simulink model "Simulation_3DOF01"  (R2024a)
settings: Solver=ode4  StartTime=initial_time  StopTime=final_time  FixedStep=timestep  RelTol=1e-3
values from neighbouring files (symbols this model uses):
  flight_path_angle_0 = flight_path_angle_0 * (pi / 180)    (= 0.0523598775598)    [Constants_3DOF.m]
  heading_angle_0 = heading_angle_0 * (pi/180)    (= 0.349065850399)    [Constants_3DOF.m]
  height_0 = 35 * 10^3    (= 35000)    [Constants_3DOF.m]
  heightsList = usAtmosphere.Z    [Constants_3DOF.m]
  latitude_0 = latitude_0 * (pi/180)    (= 0.680503875353)    [Constants_3DOF.m]
  longitude_0 = longitude_0 * (pi/180)    (= -1.26396744429)    [Constants_3DOF.m]
  mass = 161.5    [Constants_3DOF.m]
  omega_earth = 7.2921159 * 10^-5    (= 7.2921159e-05)    [Constants_3DOF.m]
  range_to_go_0 = 11112 * 10^3    (= 11112000)    [Constants_3DOF.m]
  rhoList = usAtmosphere.x_    [Constants_3DOF.m]
  speed_0 = 1500    [Constants_3DOF.m]
  temperatureList = usAtmosphere.T    [Constants_3DOF.m]
  wing_area = 0.079813    [Constants_3DOF.m]
settings Model: Creator=641893  LastModifiedBy=641893

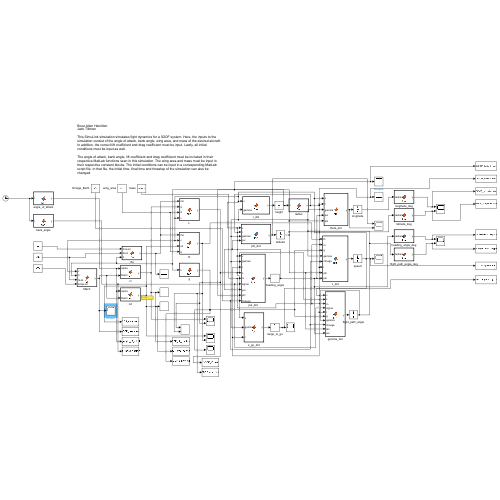
[thumbnail: Simulink's stored preview of the top-level diagram]
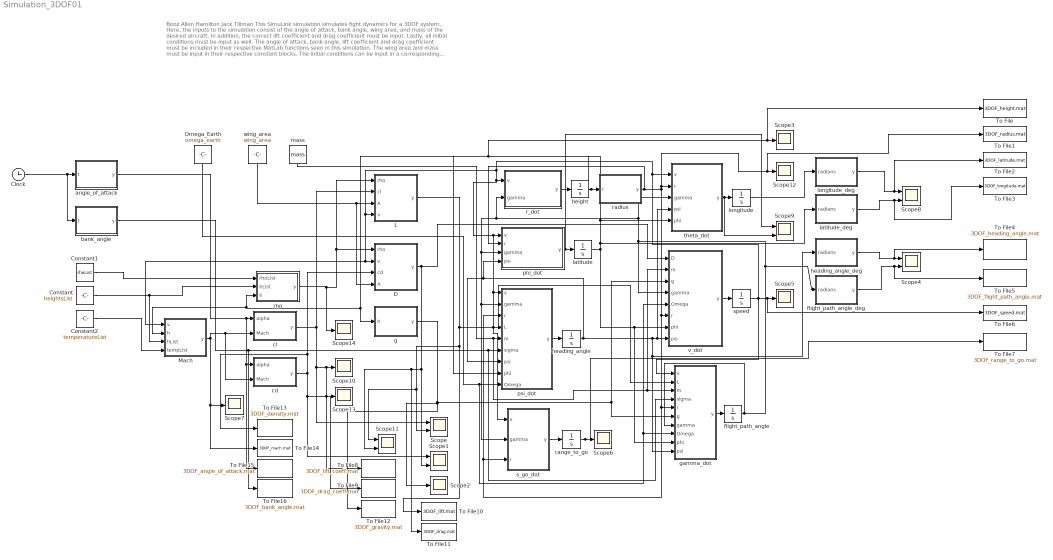
== system Simulation_3DOF01 ==
  note: Booz Allen Hamilton
      | Jack Tillman
      |
      | This SimuLink simulation simulates fight dynamics for a 3DOF system. Here, the inputs to the simulation consist of the angle of attack, bank angle, wing area, and mass of the desired aircraft. In addition, the correct lift coefficient and drag coefficient must be input. Lastly, all initial conditions must be input as well.
      |
      | The angle of attack, bank angle, lift coefficient and drag coefficient must be included in their respective MatLab functions seen in this simulation. The wing area and mass must be input in their respective constant blocks. The initial conditions can be input in a corresponding MatLab script file. In that file, the initial time, final time and timestep of the simulation can also be changed.
  Clock : Clock
  Constant : Constant  Value=heightsList
  Constant1 : Constant  Value=rhoList
  Constant2 : Constant  Value=temperatureList
  D : MATLAB Function  TreatAsAtomicUnit=on
  L : MATLAB Function  TreatAsAtomicUnit=on
  Mach : MATLAB Function  TreatAsAtomicUnit=on
  Omega_Earth : Constant  Value=omega_earth
  Scope{,1,4,8..9,11} (6 alike) : Scope  NumInputPorts=2
  Scope{2..3,5..7,10,12..14} (9 alike) : Scope
  To File : ToFile  Filename=3DOF_height.mat  MatrixName=height
  To File1 : ToFile  Filename=3DOF_radius.mat
  To File10 : ToFile  Filename=3DOF_lift.mat
  To File11 : ToFile  Filename=3DOF_drag.mat
  To File12 : ToFile  Filename=3DOF_gravity.mat
  To File13 : ToFile  Filename=3DOF_density.mat
  To File14 : ToFile  Filename=3DOF_mach.mat
  To File15 : ToFile  Filename=3DOF_angle_of_attack.mat
  To File16 : ToFile  Filename=3DOF_bank_angle.mat
  To File2 : ToFile  Filename=3DOF_latitude.mat
  To File3 : ToFile  Filename=3DOF_longitude.mat
  To File4 : ToFile  Filename=3DOF_heading_angle.mat
  To File5 : ToFile  Filename=3DOF_flight_path_angle.mat
  To File6 : ToFile  Filename=3DOF_speed.mat
  To File7 : ToFile  Filename=3DOF_range_to_go.mat
  To File8 : ToFile  Filename=3DOF_lift_coeff.mat
  To File9 : ToFile  Filename=3DOF_drag_coeff.mat
  angle_of_attack : MATLAB Function  TreatAsAtomicUnit=on
  bank_angle : MATLAB Function  TreatAsAtomicUnit=on
  cd : MATLAB Function  TreatAsAtomicUnit=on
  cl : MATLAB Function  TreatAsAtomicUnit=on
  flight_path_angle : Integrator  InitialCondition=flight_path_angle_0  ContinuousStateAttributes='flight_path_angle'
  flight_path_angle_deg : MATLAB Function  TreatAsAtomicUnit=on
  g : MATLAB Function  TreatAsAtomicUnit=on
  gamma_dot : MATLAB Function  TreatAsAtomicUnit=on
  heading_angle : Integrator  InitialCondition=heading_angle_0  ContinuousStateAttributes='heading_angle'
  heading_angle_deg : MATLAB Function  TreatAsAtomicUnit=on
  height : Integrator  InitialCondition=height_0  ContinuousStateAttributes='radius'
  latitude : Integrator  InitialCondition=latitude_0  ContinuousStateAttributes='latitude'
  latitude_deg : MATLAB Function  TreatAsAtomicUnit=on
  longitude : Integrator  InitialCondition=longitude_0  ContinuousStateAttributes='longitude'
  longitude_deg : MATLAB Function  TreatAsAtomicUnit=on
  mass : Constant  Value=mass
  phi_dot : MATLAB Function  TreatAsAtomicUnit=on
  psi_dot : MATLAB Function  TreatAsAtomicUnit=on
  r_dot : MATLAB Function  TreatAsAtomicUnit=on
  radius : MATLAB Function  TreatAsAtomicUnit=on
  range_to_go : Integrator  InitialCondition=range_to_go_0  ContinuousStateAttributes='range_to_go'
  rho : MATLAB Function  TreatAsAtomicUnit=on
  s_go_dot : MATLAB Function  TreatAsAtomicUnit=on
  speed : Integrator  InitialCondition=speed_0  ContinuousStateAttributes='velocity'
  theta_dot : MATLAB Function  TreatAsAtomicUnit=on
  v_dot : MATLAB Function  TreatAsAtomicUnit=on
  wing_area : Constant  Value=wing_area
  wires:
  rho/1(y) -> Scope14/1, D/1(rho), L/1(rho)
  cl/1(y) -> Scope/1, To File8/1, Scope10/1, L/2(cl)
  cd/1(y) -> To File13/1, D/3(cd), Scope1/1, To File9/1, Scope13/1
  wing_area/1 -> D/4(A), L/3(A)
  L/1(y) -> Scope11/1, Scope/2, To File10/1, gamma_dot/2(L), psi_dot/4(L)
  g/1(y) -> Scope2/1, To File12/1, v_dot/3(g), gamma_dot/6(g)
  mass/1 -> gamma_dot/3(m), v_dot/2(m), psi_dot/5(m)
  D/1(y) -> To File11/1, Scope11/2, Scope1/2, v_dot/1(D)
  Mach/1(y) -> cl/2(Mach), cd/2(Mach), To File14/1, Scope7/1
  Omega_Earth/1 -> psi_dot/9(Omega), gamma_dot/8(Omega), v_dot/5(Omega)
  Clock/1 -> bank_angle/1(t), angle_of_attack/1(t)
  bank_angle/1(y) -> To File16/1, psi_dot/6(sigma), gamma_dot/4(sigma)
  angle_of_attack/1(y) -> cd/1(alpha), To File15/1, cl/1(alpha)
  s_go_dot/1(y) -> range_to_go/1
  range_to_go/1 -> To File7/1, Scope6/1
  psi_dot/1(y) -> heading_angle/1
  heading_angle/1 -> psi_dot/7(psi), phi_dot/4(psi), gamma_dot/10(psi), heading_angle_deg/1(radians), v_dot/8(psi), theta_dot/4(psi)
  phi_dot/1(y) -> Scope9/1, latitude/1
  latitude/1 -> psi_dot/8(phi), theta_dot/5(phi), latitude_deg/1(radians), v_dot/7(phi), gamma_dot/9(phi)
  r_dot/1(y) -> height/1
  theta_dot/1(y) -> longitude/1, Scope9/2
  v_dot/1(y) -> speed/1
  speed/1 -> To File6/1, Scope5/1, psi_dot/1(v), s_go_dot/1(v), phi_dot/1(v), r_dot/1(v), D/2(v), Mach/1(v), L/4(v), theta_dot/1(v), gamma_dot/1(v)
  gamma_dot/1(y) -> flight_path_angle/1
  flight_path_angle/1 -> gamma_dot/7(gamma), v_dot/4(gamma), theta_dot/3(gamma), s_go_dot/2(gamma), psi_dot/2(gamma), phi_dot/3(gamma), r_dot/2(gamma), flight_path_angle_deg/1(radians)
  height/1 -> To File/1, Scope3/1, Mach/2(h), rho/3(h), g/1(h), radius/1(r)
  radius/1(y) -> phi_dot/2(r), To File1/1, Scope12/1, theta_dot/2(r), v_dot/6(r), s_go_dot/3(r), psi_dot/3(r), gamma_dot/5(r)
  longitude/1 -> longitude_deg/1(radians)
  longitude_deg/1(y) -> To File2/1, Scope8/1
  latitude_deg/1(y) -> To File3/1, Scope8/2
  heading_angle_deg/1(y) -> To File4/1, Scope4/1
  flight_path_angle_deg/1(y) -> To File5/1, Scope4/2
  Constant/1 -> Mach/3(hList), rho/2(hList)
  Constant1/1 -> rho/1(rhoList)
  Constant2/1 -> Mach/4(tempList)

== matlab function Simulation_3DOF01/D ==
  data: rho input; y output; v input; cd input; A input
function y = fcn(rho, v, cd, A)

y = 0.5 * rho * v^2 * A * cd;

== matlab function Simulation_3DOF01/g ==
  data: y output; h input
function y = fcn(h)
mu_earth = 3.96272 * 10^14;
rE = 6378140;
y = mu_earth / (rE + h)^2;

== matlab function Simulation_3DOF01/rho ==
  data: rhoList input; hList input; h input; y output
function y = fcn(rhoList, hList,h)

h = h / 10^3;

if h >= 0
    density = interp1(hList, rhoList, h);
else
    density = 0;
end


y = density;

== matlab function Simulation_3DOF01/cl ==
  data: alpha input; y output; Mach input
function y = fcn(alpha, Mach)
cl0 = -0.2317;
cl1 = 0.0513;
cl2 = 0.2945;
cl3 = -0.1028;
y = cl0 + cl1 * alpha + cl2 * exp(cl3 * Mach);

== matlab function Simulation_3DOF01/cd ==
  data: alpha input; y output; Mach input
function y = fcn(alpha, Mach)
cd0 = 0.024;
cd1 = 7.24 * 10^-4;
cd2 = 0.406;
cd3 = -0.323;
y = cd0 + cd1 * alpha^2 + cd2 * exp(cd3 * Mach);

== matlab function Simulation_3DOF01/angle_of_attack ==
  data: t input; y output
function y = fcn(t)

alpha = 19.88;
alpha = alpha * pi / 180;

y = alpha;

== matlab function Simulation_3DOF01/Mach ==
  data: v input; y output; h input; hList input; tempList input
function y = fcn(v, h, hList, tempList)

gamma = 1.4;
R = 287.05;

h = h / 10^3;

if h >= 0
    temp = interp1(hList, tempList, h);
    a = sqrt(gamma * R * temp);
    y = v/a;
else
    temp = 0;
    y = 0;
end

== matlab function Simulation_3DOF01/phi_dot ==
  data: v input; y output; r input; gamma input; psi input
function y = fcn(v, r, gamma, psi)

y = (v / r) * cos(gamma) * sin(psi);

== matlab function Simulation_3DOF01/bank_angle ==
  data: t input; y output
function y = fcn(t)

sigma = 0;
sigma = sigma * pi / 180;

y = sigma;

== matlab function Simulation_3DOF01/radius ==
  data: r input; y output
function y = fcn(r)
rE = 6378140;
radius = r + rE;
y = radius;

== matlab function Simulation_3DOF01/longitude_deg ==
  data: radians input; y output
function y = fcn(radians)
degrees = radians * (180 / pi);
y = degrees;

== matlab function Simulation_3DOF01/latitude_deg ==
  data: radians input; y output
function y = fcn(radians)
degrees = radians * (180 / pi);
y = degrees;

== matlab function Simulation_3DOF01/heading_angle_deg ==
  data: radians input; y output
function y = fcn(radians)
degrees = radians * (180 / pi);
y = degrees;

== matlab function Simulation_3DOF01/flight_path_angle_deg ==
  data: radians input; y output
function y = fcn(radians)
degrees = radians * (180 / pi);
y = degrees;

== matlab function Simulation_3DOF01/r_dot ==
  data: v input; y output; gamma input
function y = fcn(v, gamma)

y = v * sin(gamma);

== matlab function Simulation_3DOF01/theta_dot ==
  data: v input; y output; r input; gamma input; psi input; phi input
function y = fcn(v, r, gamma, psi, phi)

y = (v * cos(gamma) * cos(psi) ) / (r * cos(phi) );

== matlab function Simulation_3DOF01/v_dot ==
  data: D input; y output; m input; g input; gamma input; Omega input; r input; phi input; psi input
function y = fcn(D, m, g, gamma, Omega, r, phi, psi)

y = -(D / m) - g * sin(gamma) + Omega^2 * r * cos(phi) * ( sin(gamma) * cos(phi) - cos(gamma) * sin(phi) * cos(psi) );

== matlab function Simulation_3DOF01/gamma_dot ==
  data: v input; y output; L input; m input; sigma input; r input; g input; gamma input; Omega input; phi input; psi input
function y = fcn(v, L, m, sigma, r, g, gamma, Omega, phi, psi)

y = (1/v) * ( (L / m) * cos(sigma) + (( v^2 / r) - g) * cos(gamma) + 2 * Omega * v * cos(phi) * sin(psi) + Omega^2 * r * cos(phi) * ( cos(gamma) * cos(phi) - sin(gamma) * sin(phi) * cos(psi) ) );

== matlab function Simulation_3DOF01/psi_dot ==
  data: v input; y output; gamma input; r input; L input; m input; sigma input; psi input; phi input; Omega input
function y = fcn(v, gamma, r, L, m, sigma, psi, phi, Omega)

y = (1 / v) * ( (L / (m * cos(gamma))) * sin(sigma) + (v^2 /  r) * cos(gamma) * sin(psi) * tan(phi) - 2 * Omega * v * (tan(gamma) * cos(psi) * cos(phi) - sin(phi) ) + (Omega^2 * r / cos(gamma)) * sin(psi) * sin(phi) * cos(phi) );

== matlab function Simulation_3DOF01/s_go_dot ==
  data: v input; y output; gamma input; r input
function y = fcn(v, gamma, r)
rE = 6378140;
y = -v * cos(gamma) * rE / r;

== matlab function Simulation_3DOF01/L ==
  data: rho input; y output; cl input; A input; v input
function y = fcn(rho, cl, A, v)

y = 0.5 * rho * v^2 * A * cl;
